simulink model "TrajetoryPlanning"  (R2022b)
settings: Solver=FixedStepAuto  StartTime=0.0  StopTime=100  FixedStep=0.01  RelTol=1e-3
settings Model: Creator=Nguyễn Minh Nhựt  LastModifiedBy=Nguyễn Minh Nhựt
settings DataIOCC: ReturnWorkspaceOutputs=off

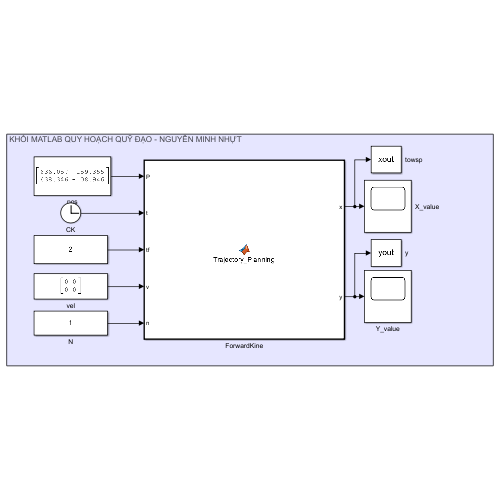
[thumbnail: Simulink's stored preview of the top-level diagram]
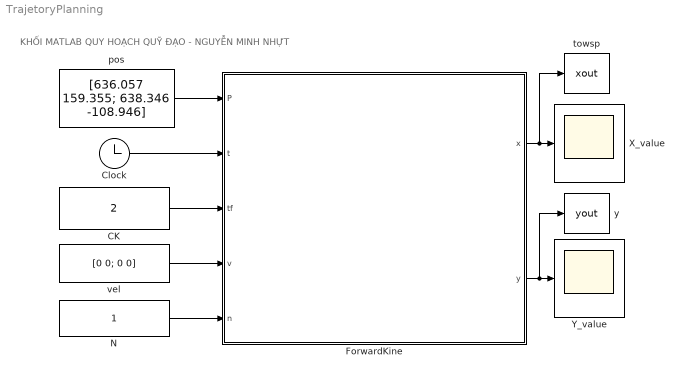
== system TrajetoryPlanning ==
  note: KHỐI MATLAB QUY HOẠCH QUỸ ĐẠO - NGUYỄN MINH NHỰT
  CK : Constant  Value=2
  Clock : Clock
      settings: Decimation=33
  ForwardKine : MATLAB Function  TreatAsAtomicUnit=on
  N : Constant
  X_value : Scope
  Y_value : Scope
  pos : Constant  Value=[636.057 159.355; 638.346 -108.946]  VectorParams1D=off
  towsp : ToWorkspace  VariableName=xout  SaveFormat=Structure With Time  SampleTime=-1
  vel : Constant  Value=[0 0; 0 0]
  y : ToWorkspace  VariableName=yout  SaveFormat=Structure With Time  SampleTime=-1
  wires:
  pos/1 -> ForwardKine/1(P)
  Clock/1 -> ForwardKine/2(t)
  N/1 -> ForwardKine/5(n)
  vel/1 -> ForwardKine/4(v)
  CK/1 -> ForwardKine/3(tf)
  ForwardKine/1(x) -> towsp/1, X_value/1
  ForwardKine/2(y) -> y/1, Y_value/1

== matlab function TrajetoryPlanning/ForwardKine ==
  data: P input; t input; x output; tf input; v input; n input; y output
%%Programmed by Nguyễn Minh Nhựt 20151143
%%Date: 11/08/2023
%%File name: Trajectory_Block
function [x, y] = Trajectory_Planning(P,t,tf,v,n)

    sum_time = n*tf; %%chu kì
    if(t < sum_time)
        tt = mod(t,tf); %% Scale lại khoảng trong thòi gian cố định
        i  = (t - mod(t,tf))/tf + 1;

        a10 = P(i,1); %x1 -> xn
        a20 = P(i,2); %y1 -> yn

        a11 = v(i,1); %v1 -> vn theo x
        a21 = v(i,2); %v1 -> vn theo y

        a12 = 3/tf^2 * (P(i+1,1) - P(i,1)) - 2/tf * v(i,1) -1/tf * v(i+1,1); %theo cot 1
        a22 = 3/tf^2 * (P(i+1,2) - P(i,2)) - 2/tf * v(i,2) -1/tf * v(i+1,2); %theo cot 2

        a13 = -2/tf^3 * (P(i+1,1)-P(i,1) + 1/tf^2 * (v(i+1,1)+ v(i,1)));
        a23 = -2/tf^3 * (P(i+1,2)-P(i,2) + 1/tf^2 * (v(i+1,2)+ v(i,2)));

        %Toa do cac diem
        x = a10 + a11*tt + a12*tt^2 + a13*tt^3
        y = a20 + a21*tt + a22*tt^2 + a23*tt^3
        hold on;
        plot(x,y); 
        plot(x,y,'*');  
    else
        x = P(length(P),1);
        y = P(length(P),2);
    end
end
